simulink model "modelAP"  (R2018b)
settings: Solver=VariableStepAuto  StartTime=0.0  StopTime=50  RelTol=1e-3
values from neighbouring files (symbols this model uses):
  A = [[k1+k2,-k2];[-k2,k2]]    [SkryptAP.m]
  B = [1 0]'    [SkryptAP.m]
  F = [[c1+c2,-c2];[-c2,c2]]    [SkryptAP.m]
settings Model: Creator=LPA4  LastModifiedBy=Kasia
settings SFSimCC: SimUseLocalCustomCode=off
settings RTWCC: RTWUseLocalCustomCode=off
settings CodeAppCC: StateflowObjectComments=on

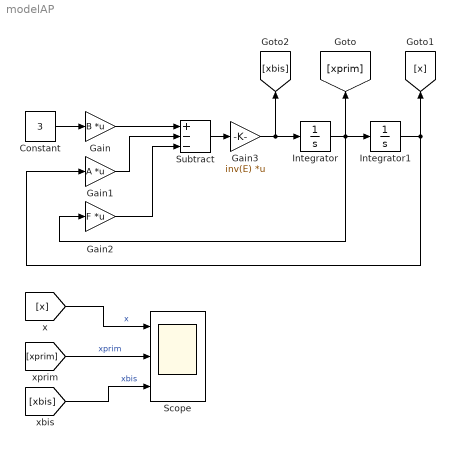
== system modelAP ==
  Constant : Constant  Value=3
  Gain : Gain  Gain=B  Multiplication=Matrix(K*u)
  Gain1 : Gain  Gain=A  Multiplication=Matrix(K*u)
  Gain2 : Gain  Gain=F  Multiplication=Matrix(K*u)
  Gain3 : Gain  Gain=inv(E)  Multiplication=Matrix(K*u)
  Integrator : Integrator  InitialCondition=[0 0]
  Integrator1 : Integrator  InitialCondition=[16 -2]
  Scope : Scope  NumInputPorts=3
  Subtract : Sum  Inputs=+--
  wires:
  Gain/1 -> Subtract/1
  Gain1/1 -> Subtract/2
  Gain2/1 -> Subtract/3
  Subtract/1 -> Gain3/1
  Gain3/1 -> Integrator/1, [xbis]
  Integrator/1 -> Integrator1/1, Gain2/1, [xprim]
  Integrator1/1 -> Gain1/1, [x]
  [x] -> Scope/1  "x"
  [xprim] -> Scope/2  "xprim"
  [xbis] -> Scope/3  "xbis"
  Constant/1 -> Gain/1
